simulink model "VMC_14Dof_2024a"  (R2024a)
settings: Solver=FixedStepDiscrete  StartTime=0.0  StopTime=10.0  FixedStep=0.001  RelTol=1e-3
InitFcn:
  | unlinear_14DOF_Parameters
undefined symbols (not defined in the file): Bf, Br, Cp_fl, Cp_fr, Cp_rl, Cp_rr, Cs_f, eta_FMotor, eta_RMotor, f, g, He, Hp, i_fa, i_ra, i_sw, I_tire, Ix, Iy, Iz, ks_f, kw, Lf, Lr, m, mb, mu, mw, r, Sampletime, Standstill_buffer, vx0, vxlim, w0
libraries: simulink x32, slpidlib x6
(part 4 of 5)

== system VMC_14Dof_2024a/Subsystem/Body/global system transform/integrator2 ==
  In : Inport
  Add : Sum
  Add1 : Sum
  Constant : Constant  Value=Sampletime  OutDataTypeStr=single
  Constant1 : Constant  Value=0  OutDataTypeStr=single
  Delay1 : Delay  DelayLength=1  InitialCondition=0
  Divide : Product  Inputs=**
  Out : Outport  VectorParamsAs1DForOutWhenUnconnected=off
  wires:
  In/1 -> Divide/1
  Constant/1 -> Divide/2
  Divide/1 -> Add/1
  Delay1/1 -> Add/2, Add1/2
  Constant1/1 -> Add1/1
  Add/1 -> Delay1/1
  Add1/1 -> Out/1

== system VMC_14Dof_2024a/Subsystem/Body/global system transform/integrator8 ==
  wz : Inport
  Add : Sum
  Add1 : Sum
  Constant : Constant  Value=Sampletime  OutDataTypeStr=single
  Constant1 : Constant  Value=0  OutDataTypeStr=single
  Delay1 : Delay  DelayLength=1  InitialCondition=0
  Divide : Product  Inputs=**
  Out : Outport  VectorParamsAs1DForOutWhenUnconnected=off
  wires:
  wz/1 -> Divide/1
  Constant/1 -> Divide/2
  Divide/1 -> Add/1
  Delay1/1 -> Add/2, Add1/2
  Constant1/1 -> Add1/1
  Add/1 -> Delay1/1
  Add1/1 -> Out/1

== system VMC_14Dof_2024a/Subsystem/Wheel/fl/integrator ==
  In : Inport
  Add : Sum
  Add1 : Sum
  Constant : Constant  Value=Sampletime  OutDataTypeStr=single
  Constant1 : Constant  Value=w0  OutDataTypeStr=single
  Delay1 : Delay  DelayLength=1  InitialCondition=0
  Divide : Product  Inputs=**
  Out : Outport  VectorParamsAs1DForOutWhenUnconnected=off
  wires:
  In/1 -> Divide/1
  Constant/1 -> Divide/2
  Divide/1 -> Add/1
  Delay1/1 -> Add/2, Add1/2
  Constant1/1 -> Add1/1
  Add/1 -> Delay1/1
  Add1/1 -> Out/1

== system VMC_14Dof_2024a/Subsystem/Wheel/fr/integrator ==
  In : Inport
  Add : Sum
  Add1 : Sum
  Constant : Constant  Value=Sampletime  OutDataTypeStr=single
  Constant1 : Constant  Value=w0  OutDataTypeStr=single
  Delay1 : Delay  DelayLength=1  InitialCondition=0
  Divide : Product  Inputs=**
  Out : Outport  VectorParamsAs1DForOutWhenUnconnected=off
  wires:
  In/1 -> Divide/1
  Constant/1 -> Divide/2
  Divide/1 -> Add/1
  Delay1/1 -> Add/2, Add1/2
  Constant1/1 -> Add1/1
  Add/1 -> Delay1/1
  Add1/1 -> Out/1

== system VMC_14Dof_2024a/Subsystem/Wheel/rl/integrator ==
  In : Inport
  Add : Sum
  Add1 : Sum
  Constant : Constant  Value=Sampletime  OutDataTypeStr=single
  Constant1 : Constant  Value=w0  OutDataTypeStr=single
  Delay1 : Delay  DelayLength=1  InitialCondition=0
  Divide : Product  Inputs=**
  Out : Outport  VectorParamsAs1DForOutWhenUnconnected=off
  wires:
  In/1 -> Divide/1
  Constant/1 -> Divide/2
  Divide/1 -> Add/1
  Delay1/1 -> Add/2, Add1/2
  Constant1/1 -> Add1/1
  Add/1 -> Delay1/1
  Add1/1 -> Out/1

== system VMC_14Dof_2024a/Subsystem/Wheel/rr/integrator ==
  In : Inport
  Add : Sum
  Add1 : Sum
  Constant : Constant  Value=Sampletime  OutDataTypeStr=single
  Constant1 : Constant  Value=w0  OutDataTypeStr=single
  Delay1 : Delay  DelayLength=1  InitialCondition=0
  Divide : Product  Inputs=**
  Out : Outport  VectorParamsAs1DForOutWhenUnconnected=off
  wires:
  In/1 -> Divide/1
  Constant/1 -> Divide/2
  Divide/1 -> Add/1
  Delay1/1 -> Add/2, Add1/2
  Constant1/1 -> Add1/1
  Add/1 -> Delay1/1
  Add1/1 -> Out/1

== system VMC_14Dof_2024a/Subsystem/alpha_lamda/alpha/fl ==
  vx : Inport
  vy : Inport  Port=2
  wz : Inport  Port=3
  delta_fl : Inport  Port=4
  Add2 : Sum
  Add3 : Sum  Inputs=+-
  Add4 : Sum  Inputs=-+
  Divide : Product  Inputs=/*
  Gain3 : Gain  Gain=Lf
  Gain4 : Gain  Gain=0.5*Bf
  Trigonometric Function : Trigonometry  Operator=atan
  alpha_fl : Outport  VectorParamsAs1DForOutWhenUnconnected=off
  wires:
  Gain3/1 -> Add2/2
  Gain4/1 -> Add3/2
  Add2/1 -> Divide/2
  Add3/1 -> Divide/1
  Divide/1 -> Trigonometric Function/1
  Trigonometric Function/1 -> Add4/1
  vx/1 -> Add3/1
  delta_fl/1 -> Add4/2
  vy/1 -> Add2/1
  Add4/1 -> alpha_fl/1
  wz/1 -> Gain4/1, Gain3/1

== system VMC_14Dof_2024a/Subsystem/alpha_lamda/alpha/fr ==
  vx : Inport
  vy : Inport  Port=2
  wz : Inport  Port=3
  delta_fr : Inport  Port=4
  Add2 : Sum
  Add3 : Sum
  Add4 : Sum  Inputs=-+
  Divide : Product  Inputs=/*
  Gain3 : Gain  Gain=Lf
  Gain4 : Gain  Gain=0.5*Bf
  Trigonometric Function : Trigonometry  Operator=atan
  alpha_fr : Outport  VectorParamsAs1DForOutWhenUnconnected=off
  wires:
  Gain4/1 -> Add3/2
  wz/1 -> Gain3/1, Gain4/1
  Add4/1 -> alpha_fr/1
  vy/1 -> Add2/1
  delta_fr/1 -> Add4/2
  vx/1 -> Add3/1
  Trigonometric Function/1 -> Add4/1
  Divide/1 -> Trigonometric Function/1
  Add3/1 -> Divide/1
  Add2/1 -> Divide/2
  Gain3/1 -> Add2/2

== system VMC_14Dof_2024a/Subsystem/alpha_lamda/alpha/rl ==
  vx : Inport
  vy : Inport  Port=2
  wz : Inport  Port=3
  Add2 : Sum  Inputs=+-
  Add3 : Sum  Inputs=+-
  Divide : Product  Inputs=/*
  Gain1 : Gain  Gain=-1
  Gain3 : Gain  Gain=Lr
  Gain4 : Gain  Gain=0.5*Br
  Trigonometric Function : Trigonometry  Operator=atan
  alpha_rl : Outport  VectorParamsAs1DForOutWhenUnconnected=off
  wires:
  Gain1/1 -> alpha_rl/1
  Gain4/1 -> Add3/2
  Trigonometric Function/1 -> Gain1/1
  wz/1 -> Gain3/1, Gain4/1
  vy/1 -> Add2/1
  vx/1 -> Add3/1
  Divide/1 -> Trigonometric Function/1
  Add3/1 -> Divide/1
  Add2/1 -> Divide/2
  Gain3/1 -> Add2/2

== system VMC_14Dof_2024a/Subsystem/alpha_lamda/alpha/rr ==
  vx : Inport
  vy : Inport  Port=2
  wz : Inport  Port=3
  Add2 : Sum  Inputs=+-
  Add3 : Sum
  Divide : Product  Inputs=/*
  Gain2 : Gain  Gain=-1
  Gain3 : Gain  Gain=Lr
  Gain4 : Gain  Gain=0.5*Br
  Trigonometric Function : Trigonometry  Operator=atan
  alpha_rr : Outport  VectorParamsAs1DForOutWhenUnconnected=off
  wires:
  Gain2/1 -> alpha_rr/1
  Gain4/1 -> Add3/2
  Gain3/1 -> Add2/2
  Add2/1 -> Divide/2
  Add3/1 -> Divide/1
  Divide/1 -> Trigonometric Function/1
  vx/1 -> Add3/1
  vy/1 -> Add2/1
  wz/1 -> Gain4/1, Gain3/1
  Trigonometric Function/1 -> Gain2/1

== system VMC_14Dof_2024a/Subsystem/alpha_lamda/lamda/fl ==
  w_fl : Inport
  wz : Inport  Port=2
  vx : Inport  Port=3
  vy : Inport  Port=4
  delta_fl : Inport  Port=5
  Add1 : Sum  Inputs=-+
  Add2 : Sum
  Add3 : Sum
  Add4 : Sum  Inputs=+-
  Constant1 : Constant  Value=r  OutDataTypeStr=single
  Divide1 : Product  Inputs=**
  Divide2 : Product  Inputs=**
  Divide3 : Product  Inputs=**
  Divide4 : Product  Inputs=/*
  Divide5 : Product  Inputs=*/
  Fcn1 : Fcn  Expr=u+(u==0)*eps
  Gain2 : Gain  Gain=0.5*Bf
  Gain3 : Gain  Gain=Lf
  Saturation : Saturate  UpperLimit=1  LowerLimit=-1
  Switch : Switch  Criteria=u2 > Threshold  SaturateOnIntegerOverflow=off  InputSameDT=off
  Trigonometric Function1 : Trigonometry
  Trigonometric Function2 : Trigonometry  Operator=cos
  lamda_fl : Outport  VectorParamsAs1DForOutWhenUnconnected=off
  wires:
  Saturation/1 -> lamda_fl/1
  Divide3/1 -> Fcn1/1, Add4/1  "w*I_tire"
  Constant1/1 -> Divide3/2
  w_fl/1 -> Divide3/1
  Divide2/1 -> Add3/2
  Divide1/1 -> Add3/1
  Trigonometric Function1/1 -> Divide2/2
  Add2/1 -> Divide2/1
  Gain3/1 -> Add2/1
  vy/1 -> Add2/2
  Trigonometric Function2/1 -> Divide1/2
  delta_fl/1 -> Trigonometric Function1/1, Trigonometric Function2/1
  Add1/1 -> Divide1/1
  wz/1 -> Gain2/1, Gain3/1
  Gain2/1 -> Add1/1
  vx/1 -> Add1/2
  Fcn1/1 -> Divide4/1
  Divide5/1 -> Switch/3
  Divide4/1 -> Switch/1
  Add4/1 -> Divide5/1, Divide4/2, Switch/2
  Add3/1 -> Divide5/2, Add4/2  "Vwx_fl"
  Switch/1 -> Saturation/1

== system VMC_14Dof_2024a/Subsystem/alpha_lamda/lamda/fr ==
  w_fr : Inport
  wz : Inport  Port=2
  vx : Inport  Port=3
  vy : Inport  Port=4
  delta_fr : Inport  Port=5
  Add1 : Sum
  Add2 : Sum
  Add3 : Sum
  Add4 : Sum  Inputs=+-
  Constant1 : Constant  Value=r  OutDataTypeStr=single
  Divide1 : Product  Inputs=**
  Divide2 : Product  Inputs=**
  Divide3 : Product  Inputs=**
  Divide4 : Product  Inputs=/*
  Divide5 : Product  Inputs=*/
  Fcn1 : Fcn  Expr=u+(u==0)*eps
  Gain2 : Gain  Gain=0.5*Bf
  Gain3 : Gain  Gain=Lf
  Saturation : Saturate  UpperLimit=1  LowerLimit=-1
  Switch : Switch  Criteria=u2 > Threshold  SaturateOnIntegerOverflow=off  InputSameDT=off
  Trigonometric Function1 : Trigonometry
  Trigonometric Function2 : Trigonometry  Operator=cos
  lamda_fr : Outport  VectorParamsAs1DForOutWhenUnconnected=off
  wires:
  Switch/1 -> Saturation/1
  Add3/1 -> Add4/2, Divide5/2  "Vwx_fr"
  Add4/1 -> Switch/2, Divide4/2, Divide5/1
  Divide4/1 -> Switch/1
  Divide5/1 -> Switch/3
  Fcn1/1 -> Divide4/1
  Divide3/1 -> Add4/1, Fcn1/1  "w*I_tire"
  Constant1/1 -> Divide3/2
  w_fr/1 -> Divide3/1
  Divide2/1 -> Add3/2
  Divide1/1 -> Add3/1
  Trigonometric Function1/1 -> Divide2/2
  Add2/1 -> Divide2/1
  Gain3/1 -> Add2/1
  vy/1 -> Add2/2
  Trigonometric Function2/1 -> Divide1/2
  delta_fr/1 -> Trigonometric Function1/1, Trigonometric Function2/1
  Add1/1 -> Divide1/1
  wz/1 -> Gain2/1, Gain3/1
  Gain2/1 -> Add1/1
  vx/1 -> Add1/2
  Saturation/1 -> lamda_fr/1

== system VMC_14Dof_2024a/Subsystem/alpha_lamda/lamda/rl ==
  w_rl : Inport
  wz : Inport  Port=2
  vx : Inport  Port=3
  Add1 : Sum  Inputs=-+
  Add4 : Sum  Inputs=+-
  Constant1 : Constant  Value=r  OutDataTypeStr=single
  Divide3 : Product  Inputs=**
  Divide4 : Product  Inputs=/*
  Divide5 : Product  Inputs=*/
  Fcn1 : Fcn  Expr=u+(u==0)*eps
  Gain2 : Gain  Gain=0.5*Br
  Saturation : Saturate  UpperLimit=1  LowerLimit=-1
  Switch : Switch  Criteria=u2 > Threshold  SaturateOnIntegerOverflow=off  InputSameDT=off
  lamda_rl : Outport  VectorParamsAs1DForOutWhenUnconnected=off
  wires:
  Switch/1 -> Saturation/1
  Add1/1 -> Add4/2, Divide5/2
  Add4/1 -> Switch/2, Divide4/2, Divide5/1
  Divide4/1 -> Switch/1
  Divide5/1 -> Switch/3
  Fcn1/1 -> Divide4/1
  Divide3/1 -> Add4/1, Fcn1/1  "w*I_tire"
  Constant1/1 -> Divide3/2
  w_rl/1 -> Divide3/1
  wz/1 -> Gain2/1
  Gain2/1 -> Add1/1
  vx/1 -> Add1/2
  Saturation/1 -> lamda_rl/1

== system VMC_14Dof_2024a/Subsystem/alpha_lamda/lamda/rr ==
  w_rr : Inport
  wz : Inport  Port=2
  vx : Inport  Port=3
  Add1 : Sum
  Add4 : Sum  Inputs=+-
  Constant1 : Constant  Value=r  OutDataTypeStr=single
  Divide3 : Product  Inputs=**
  Divide4 : Product  Inputs=/*
  Divide5 : Product  Inputs=*/
  Fcn1 : Fcn  Expr=u+(u==0)*eps
  Gain2 : Gain  Gain=0.5*Br
  Saturation : Saturate  UpperLimit=1  LowerLimit=-1
  Switch : Switch  Criteria=u2 > Threshold  SaturateOnIntegerOverflow=off  InputSameDT=off
  lamda_rr : Outport  VectorParamsAs1DForOutWhenUnconnected=off
  wires:
  Add1/1 -> Add4/2, Divide5/2  "Vwx_rr"
  Add4/1 -> Switch/2, Divide4/2, Divide5/1
  Divide4/1 -> Switch/1
  Divide5/1 -> Switch/3
  Fcn1/1 -> Divide4/1
  Divide3/1 -> Add4/1, Fcn1/1  "w*I_tire"
  vx/1 -> Add1/2
  Gain2/1 -> Add1/1
  wz/1 -> Gain2/1
  w_rr/1 -> Divide3/1
  Constant1/1 -> Divide3/2
  Switch/1 -> Saturation/1
  Saturation/1 -> lamda_rr/1

== system VMC_14Dof_2024a/Subsystem1/Traction_Control/LSD_Enable/LSD_EnableFL ==
  BrkDmd : Inport
  WhlSpdActlFL : Inport  Port=2
  WhlSpdRefFL : Inport  Port=3
  Compare To Constant1 : simulink/Logic and Bit Operations/Compare To Constant  relop=<  const=0.1  OutDataTypeStr=boolean
  Compare To Constant3 : simulink/Logic and Bit Operations/Compare To Constant  relop=>=  const=2  OutDataTypeStr=boolean
  Logical Operator : Logic  Inputs=3  AllPortsSameDT=off  OutDataTypeStr=boolean
  SlipJudge : simulink/Logic and Bit Operations/Compare To Constant  relop=>=  const=0.1  OutDataTypeStr=boolean
  LSD_EnableFL : Outport  VectorParamsAs1DForOutWhenUnconnected=off
  wires:
  WhlSpdActlFL/1 -> Compare To Constant3/1
  WhlSpdRefFL/1 -> SlipJudge/1  "SlipRateFL"
  Compare To Constant1/1 -> Logical Operator/1
  BrkDmd/1 -> Compare To Constant1/1
  Logical Operator/1 -> LSD_EnableFL/1  "LSD_EnableFL"
  Compare To Constant3/1 -> Logical Operator/2
  SlipJudge/1 -> Logical Operator/3

== system VMC_14Dof_2024a/Subsystem1/Traction_Control/LSD_Enable/LSD_EnableFR ==
  BrkDmd : Inport
  WhlSpdActlFR : Inport  Port=2
  WhlSpdRefFR : Inport  Port=3
  Compare To Constant1 : simulink/Logic and Bit Operations/Compare To Constant  relop=<  const=0.1  OutDataTypeStr=boolean
  Compare To Constant3 : simulink/Logic and Bit Operations/Compare To Constant  relop=>=  const=2  OutDataTypeStr=boolean
  Logical Operator : Logic  Inputs=3  AllPortsSameDT=off  OutDataTypeStr=boolean
  SlipJudge : simulink/Logic and Bit Operations/Compare To Constant  relop=>=  const=0.1  OutDataTypeStr=boolean
  LSD_EnableFL : Outport  VectorParamsAs1DForOutWhenUnconnected=off
  wires:
  SlipJudge/1 -> Logical Operator/3
  Compare To Constant3/1 -> Logical Operator/2
  Logical Operator/1 -> LSD_EnableFL/1  "LSD_EnableFL"
  BrkDmd/1 -> Compare To Constant1/1
  Compare To Constant1/1 -> Logical Operator/1
  WhlSpdRefFR/1 -> SlipJudge/1  "SlipRateFR"
  WhlSpdActlFR/1 -> Compare To Constant3/1

== system VMC_14Dof_2024a/Subsystem1/Traction_Control/LSD_Enable/LSD_EnableRL ==
  BrkDmd : Inport
  WhlSpdActlRL : Inport  Port=2
  WhlSpdRefRL : Inport  Port=3
  Compare To Constant1 : simulink/Logic and Bit Operations/Compare To Constant  relop=<  const=0.1  OutDataTypeStr=boolean
  Compare To Constant3 : simulink/Logic and Bit Operations/Compare To Constant  relop=>=  const=2  OutDataTypeStr=boolean
  Logical Operator : Logic  Inputs=3  AllPortsSameDT=off  OutDataTypeStr=boolean
  SlipJudge : simulink/Logic and Bit Operations/Compare To Constant  relop=>=  const=0.1  OutDataTypeStr=boolean
  LSD_EnableFL : Outport  VectorParamsAs1DForOutWhenUnconnected=off
  wires:
  WhlSpdActlRL/1 -> Compare To Constant3/1
  WhlSpdRefRL/1 -> SlipJudge/1  "SlipRateRL"
  Compare To Constant1/1 -> Logical Operator/1
  BrkDmd/1 -> Compare To Constant1/1
  Logical Operator/1 -> LSD_EnableFL/1  "LSD_EnableFL"
  Compare To Constant3/1 -> Logical Operator/2
  SlipJudge/1 -> Logical Operator/3

== system VMC_14Dof_2024a/Subsystem1/Traction_Control/LSD_Enable/LSD_EnableRR  ==
  BrkDmd : Inport
  WhlSpdActlRR : Inport  Port=2
  WhlSpdRefRR : Inport  Port=3
  Compare To Constant1 : simulink/Logic and Bit Operations/Compare To Constant  relop=<  const=0.1  OutDataTypeStr=boolean
  Compare To Constant3 : simulink/Logic and Bit Operations/Compare To Constant  relop=>=  const=2  OutDataTypeStr=boolean
  Logical Operator : Logic  Inputs=3  AllPortsSameDT=off  OutDataTypeStr=boolean
  SlipJudge : simulink/Logic and Bit Operations/Compare To Constant  relop=>=  const=0.1  OutDataTypeStr=boolean
  LSD_EnableFL : Outport  VectorParamsAs1DForOutWhenUnconnected=off
  wires:
  SlipJudge/1 -> Logical Operator/3
  Compare To Constant3/1 -> Logical Operator/2
  Logical Operator/1 -> LSD_EnableFL/1  "LSD_EnableFL"
  BrkDmd/1 -> Compare To Constant1/1
  Compare To Constant1/1 -> Logical Operator/1
  WhlSpdRefRR/1 -> SlipJudge/1  "SlipRateRR"
  WhlSpdActlRR/1 -> Compare To Constant3/1

== system VMC_14Dof_2024a/Subsystem1/Traction_Control/LimitedSlipDifferential/LSD_Ctrl ==
  Vehicle_States : Inport
  LSD_Enable : Inport  Port=2
  Bus Creator{,1..3} (4 alike) : BusCreator  Inputs=3
  Bus Selector : BusSelector  OutputSignals=Wheel.Ref_WheelSpeed_Array_radps,Vehicle_Static_Parameter.Gear_Ratio_NA,Torque_Demand.MotorSpeed_Array_rpm
  Constant : Constant  Value=30 / pi  OutDataTypeStr=single
  Demux : Demux
  Demux1 : Demux
  Demux2 : Demux
  Divide : Product  Inputs=***  OutDataTypeStr=single
  LSD_CtrlFL : Outport
  LSD_CtrlFR : Outport  Port=2
  LSD_CtrlRL : Outport  Port=3
  LSD_CtrlRR : Outport  Port=4
  wires:
  Constant/1 -> Divide/3
  Demux2/4 -> Bus Creator3/1  "MotSpdRefByrpmRR"
  Divide/1 -> Demux2/1  "MotSpdRefbyrpm"
  Demux2/1 -> Bus Creator/1  "MotSpdRefByrpmFL"
  Demux2/2 -> Bus Creator1/1  "MotSpdRefByrpmFR"
  Demux2/3 -> Bus Creator2/1  "MotSpdRefByrpmRL"
  Demux1/4 -> Bus Creator3/2  "MotSpdActlByrpmRR"
  Demux1/2 -> Bus Creator1/2  "MotSpdActlByrpmFR"
  Demux1/3 -> Bus Creator2/2  "MotSpdActlByrpmRL"
  Demux1/1 -> Bus Creator/2  "MotSpdActlByrpmFL"
  Demux/1 -> Bus Creator/3  "LSD_EnableFL"
  Demux/2 -> Bus Creator1/3  "LSD_EnableFR"
  Demux/3 -> Bus Creator2/3  "LSD_EnableRL"
  Demux/4 -> Bus Creator3/3  "LSD_EnableRR"
  Bus Creator/1 -> LSD_CtrlFL/1  "LSD_CtrlFL"
  Bus Creator1/1 -> LSD_CtrlFR/1  "LSD_CtrlFR"
  Bus Creator2/1 -> LSD_CtrlRL/1  "LSD_CtrlRL"
  Bus Creator3/1 -> LSD_CtrlRR/1  "LSD_CtrlRR"
  Bus Selector/1 -> Divide/1  "<Ref_WheelSpeed_Array_radps>"
  LSD_Enable/1 -> Demux/1
  Bus Selector/3 -> Demux1/1  "<MotorSpeed_Array_rpm>"
  Vehicle_States/1 -> Bus Selector/1
  Bus Selector/2 -> Divide/2  "<Gear_Ratio_NA>"

== system VMC_14Dof_2024a/Subsystem1/Traction_Control/LimitedSlipDifferential/PID_CtrlFL ==
  LSD_CtrlFL : Inport
  EDS_TrqFL : Inport  Port=2
  PID_Setting : Inport  Port=3
  Add1 : Sum  AccumDataTypeStr=single
  Bus Selector : BusSelector  OutputSignals=MotSpdRefByrpmFL,MotSpdActlByrpmFL,LSD_EnableFL
  Demux : Demux  Outputs=5
  Gain : Gain  Gain=0.001  ParamDataTypeStr=single  OutDataTypeStr=single
  PID Controller : slpidlib/PID Controller  Controller=PID  Form=Parallel  TimeDomain=Discrete-time  UseExternalTs=off  SampleTime=-1  IntegratorMethod=Forward Euler  FilterMethod=Forward Euler  ControllerParametersSource=external  P=500  I=0  UseKiTs=off  D=0  UseExternalDerivativeSource=off  N=100  UseFilter=on  TunerSelectOption=Transfer Function Based (PID Tuner App)  InitialConditionSource=internal  InitialConditionForIntegrator=0  InitialConditionForFilter=0  DifferentiatorICPrevScaledInput=0  ExternalReset=rising  TrackingMode=off  Kt=1  LimitOutput=off  SatLimitsSource=internal  UpperSaturationLimit=inf  LowerSaturationLimit=-inf  LinearizeAsGain=on  AntiWindupMode=none  Kb=1  LimitIntegrator=off  UpperIntegratorSaturationLimit=inf  LowerIntegratorSaturationLimit=-inf  PGainOutDataTypeStr=single  PProdOutDataTypeStr=single  POutMin=[]  POutMax=[]  IGainOutDataTypeStr=single  IProdOutDataTypeStr=single  IOutMin=[]  IOutMax=[]  DGainOutDataTypeStr=single  DProdOutDataTypeStr=single  DOutMin=[]  DOutMax=[]  NGainOutDataTypeStr=single  NProdOutDataTypeStr=single  NOutMin=[]  NOutMax=[]  SumOutDataTypeStr=single  SumOutMin=[]  SumOutMax=[]  SaturationOutMin=[]  SaturationOutMax=[]  PParamMin=[]  PParamMax=[]  IParamMin=[]  IParamMax=[]  DParamMin=[]  DParamMax=[]  NParamMin=[]  NParamMax=[]  KbParamMin=[]  KbParamMax=[]  KtParamMin=[]  KtParamMax=[]  KbOutMin=[]  KbOutMax=[]  KtOutMin=[]  KtOutMax=[]  IntegratorOutMin=[]  IntegratorOutMax=[]  FilterOutMin=[]  FilterOutMax=[]  SumI1OutMin=[]  SumI1OutMax=[]  SumI2OutMin=[]  SumI2OutMax=[]  SumI3OutMin=[]  SumI3OutMax=[]  SumI4OutMin=[]  SumI4OutMax=[]  SumDOutMin=[]  SumDOutMax=[]  DifferentiatorOutMin=[]  DifferentiatorOutMax=[]  FilterDiffOutCoefMin=[]  FilterDiffOutCoefMax=[]  ReciprocalOutMin=[]  ReciprocalOutMax=[]  SumDenOutMin=[]  SumDenOutMax=[]  SumNumOutMin=[]  SumNumOutMax=[]  DivideOutMin=[]  DivideOutMax=[]  UdiffTsProdOutMin=[]  UdiffTsProdOutMax=[]  NTsProdOutMin=[]  NTsProdOutMax=[]  UintegralTsProdOutMin=[]  UintegralTsProdOutMax=[]  UngainTsProdOutMin=[]  UngainTsProdOutMax=[]  ClampingZeroOutDataTypeStr=Inherit: Inherit via back propagation  ClampingZeroOutMin=[]  ClampingZeroOutMax=[]  FilterDenConstantOutDataTypeStr=Inherit: Inherit via back propagation  FilterDenConstantOutMin=[]  FilterDenConstantOutMax=[]  PCopyOutDataTypeStr=Inherit: Inherit via back propagation  PCopyOutMin=[]  PCopyOutMax=[]  NCopyOutDataTypeStr=Inherit: Inherit via back propagation  NCopyOutMin=[]  NCopyOutMax=[]  IntegratorContinuousStateAttributes=''  IntegratorStateMustResolveToSignalObject=off  IntegratorRTWStateStorageClass=Auto  FilterContinuousStateAttributes=''  FilterStateMustResolveToSignalObject=off  FilterRTWStateStorageClass=Auto  ParallelPVariant=ExternalParameters  IdealPVariant=Disabled  IVariant=ExternalParameters  DVariant=ExternalParameters  IntegratorVariant=Discrete  SatVariant=Disabled  AWVariant=Passthrough  PCopyVariant=Disabled  TRVariant=Disabled  FdbkBlocksVariant=Forward  IdealPFdbkVariant=Disabled  SatFdbkVariant=Disabled  DerivativeFilterVariant=ForwardEulerFilter  NVariant=ExternalParameters  NCopyVariant=Disabled  FilterICVariant=InternalICsFilter  IntegratorICVariant=InternalICs  ExternalResetVariant=ExternalReset  TRSumVariant=Passthrough  SumFdbkVariant=Disabled  SumVariant=Sum_PID  TsampFilterVariant=InternalTs  TsampNgainVariant=Passthrough  TsampIntegralVariant=Disabled_SignalSpec  ExternalSaturationOutDataTypeStr=Inherit: Same as second input  DerivativeSourceVariant=ErrorSignal
  Saturation1 : Saturate  UpperLimit=0  LowerLimit=-10
  SpdDiffFL : Sum  Inputs=+-  OutDataTypeStr=single  AccumDataTypeStr=single
  Switch : Switch  Criteria=u2 > Threshold  OutDataTypeStr=single  SaturateOnIntegerOverflow=off  InputSameDT=off
  LSD_TrqFL : Outport  VectorParamsAs1DForOutWhenUnconnected=off
  wires:
  Add1/1 -> Switch/1  "LSDTrqFL"
  EDS_TrqFL/1 -> Add1/2, Switch/3
  LSD_CtrlFL/1 -> Bus Selector/1
  Bus Selector/1 -> SpdDiffFL/1  "<MotSpdRefByrpmFL>"
  Bus Selector/2 -> SpdDiffFL/2  "<MotSpdActlByrpmFL>"
  Bus Selector/3 -> Switch/2  "<LSD_EnableFL>"
  Switch/1 -> LSD_TrqFL/1  "LSD_TrqFL"
  Demux/4 -> PID Controller/5  "N"
  Demux/1 -> PID Controller/2  "P"
  PID Controller/1 -> Saturation1/1  "TrqModFL"
  Demux/2 -> PID Controller/3  "I"
  Demux/3 -> PID Controller/4  "D"
  Demux/5 -> PID Controller/6  "PID_Reset"
  PID_Setting/1 -> Demux/1
  Gain/1 -> PID Controller/1  "SpdDiffFLScaled"
  SpdDiffFL/1 -> Gain/1  "SpdDiffFL"
  Saturation1/1 -> Add1/1

== system VMC_14Dof_2024a/Subsystem1/Traction_Control/LimitedSlipDifferential/PID_CtrlFR ==
  LSD_CtrlFR : Inport
  EDS_TrqFR : Inport  Port=2
  PID_Setting : Inport  Port=3
  Add1 : Sum  AccumDataTypeStr=single
  Bus Selector : BusSelector  OutputSignals=MotSpdRefByrpmFR,MotSpdActlByrpmFR,LSD_EnableFR
  Demux : Demux  Outputs=5
  Gain : Gain  Gain=0.001  ParamDataTypeStr=single  OutDataTypeStr=single
  PID Controller : slpidlib/PID Controller  Controller=PID  Form=Parallel  TimeDomain=Discrete-time  UseExternalTs=off  SampleTime=-1  IntegratorMethod=Forward Euler  FilterMethod=Forward Euler  ControllerParametersSource=external  P=500  I=0  UseKiTs=off  D=0  UseExternalDerivativeSource=off  N=100  UseFilter=on  TunerSelectOption=Transfer Function Based (PID Tuner App)  InitialConditionSource=internal  InitialConditionForIntegrator=0  InitialConditionForFilter=0  DifferentiatorICPrevScaledInput=0  ExternalReset=rising  TrackingMode=off  Kt=1  LimitOutput=off  SatLimitsSource=internal  UpperSaturationLimit=inf  LowerSaturationLimit=-inf  LinearizeAsGain=on  AntiWindupMode=none  Kb=1  LimitIntegrator=off  UpperIntegratorSaturationLimit=inf  LowerIntegratorSaturationLimit=-inf  PGainOutDataTypeStr=single  PProdOutDataTypeStr=single  POutMin=[]  POutMax=[]  IGainOutDataTypeStr=single  IProdOutDataTypeStr=single  IOutMin=[]  IOutMax=[]  DGainOutDataTypeStr=single  DProdOutDataTypeStr=single  DOutMin=[]  DOutMax=[]  NGainOutDataTypeStr=single  NProdOutDataTypeStr=single  NOutMin=[]  NOutMax=[]  SumOutDataTypeStr=single  SumOutMin=[]  SumOutMax=[]  SaturationOutMin=[]  SaturationOutMax=[]  PParamMin=[]  PParamMax=[]  IParamMin=[]  IParamMax=[]  DParamMin=[]  DParamMax=[]  NParamMin=[]  NParamMax=[]  KbParamMin=[]  KbParamMax=[]  KtParamMin=[]  KtParamMax=[]  KbOutMin=[]  KbOutMax=[]  KtOutMin=[]  KtOutMax=[]  IntegratorOutMin=[]  IntegratorOutMax=[]  FilterOutMin=[]  FilterOutMax=[]  SumI1OutMin=[]  SumI1OutMax=[]  SumI2OutMin=[]  SumI2OutMax=[]  SumI3OutMin=[]  SumI3OutMax=[]  SumI4OutMin=[]  SumI4OutMax=[]  SumDOutMin=[]  SumDOutMax=[]  DifferentiatorOutMin=[]  DifferentiatorOutMax=[]  FilterDiffOutCoefMin=[]  FilterDiffOutCoefMax=[]  ReciprocalOutMin=[]  ReciprocalOutMax=[]  SumDenOutMin=[]  SumDenOutMax=[]  SumNumOutMin=[]  SumNumOutMax=[]  DivideOutMin=[]  DivideOutMax=[]  UdiffTsProdOutMin=[]  UdiffTsProdOutMax=[]  NTsProdOutMin=[]  NTsProdOutMax=[]  UintegralTsProdOutMin=[]  UintegralTsProdOutMax=[]  UngainTsProdOutMin=[]  UngainTsProdOutMax=[]  ClampingZeroOutDataTypeStr=Inherit: Inherit via back propagation  ClampingZeroOutMin=[]  ClampingZeroOutMax=[]  FilterDenConstantOutDataTypeStr=Inherit: Inherit via back propagation  FilterDenConstantOutMin=[]  FilterDenConstantOutMax=[]  PCopyOutDataTypeStr=Inherit: Inherit via back propagation  PCopyOutMin=[]  PCopyOutMax=[]  NCopyOutDataTypeStr=Inherit: Inherit via back propagation  NCopyOutMin=[]  NCopyOutMax=[]  IntegratorContinuousStateAttributes=''  IntegratorStateMustResolveToSignalObject=off  IntegratorRTWStateStorageClass=Auto  FilterContinuousStateAttributes=''  FilterStateMustResolveToSignalObject=off  FilterRTWStateStorageClass=Auto  ParallelPVariant=ExternalParameters  IdealPVariant=Disabled  IVariant=ExternalParameters  DVariant=ExternalParameters  IntegratorVariant=Discrete  SatVariant=Disabled  AWVariant=Passthrough  PCopyVariant=Disabled  TRVariant=Disabled  FdbkBlocksVariant=Forward  IdealPFdbkVariant=Disabled  SatFdbkVariant=Disabled  DerivativeFilterVariant=ForwardEulerFilter  NVariant=ExternalParameters  NCopyVariant=Disabled  FilterICVariant=InternalICsFilter  IntegratorICVariant=InternalICs  ExternalResetVariant=ExternalReset  TRSumVariant=Passthrough  SumFdbkVariant=Disabled  SumVariant=Sum_PID  TsampFilterVariant=InternalTs  TsampNgainVariant=Passthrough  TsampIntegralVariant=Disabled_SignalSpec  ExternalSaturationOutDataTypeStr=Inherit: Same as second input  DerivativeSourceVariant=ErrorSignal
  Saturation1 : Saturate  UpperLimit=0  LowerLimit=-10
  SpdDiffFR : Sum  Inputs=+-  OutDataTypeStr=single  AccumDataTypeStr=single
  Switch : Switch  Criteria=u2 > Threshold  OutDataTypeStr=single  SaturateOnIntegerOverflow=off  InputSameDT=off
  LSD_TrqFR : Outport  VectorParamsAs1DForOutWhenUnconnected=off
  wires:
  Add1/1 -> Switch/1  "LSDTrqFR"
  LSD_CtrlFR/1 -> Bus Selector/1
  Switch/1 -> LSD_TrqFR/1  "LSD_TrqFR"
  Bus Selector/3 -> Switch/2  "<LSD_EnableFR>"
  EDS_TrqFR/1 -> Add1/2, Switch/3
  PID Controller/1 -> Saturation1/1  "TrqModFR"
  Bus Selector/2 -> SpdDiffFR/2  "<MotSpdActlByrpmFR>"
  Demux/3 -> PID Controller/4  "D"
  Demux/2 -> PID Controller/3  "I"
  PID_Setting/1 -> Demux/1
  Demux/5 -> PID Controller/6  "PID_Reset"
  Gain/1 -> PID Controller/1  "SpdDiffFRScaled"
  Demux/4 -> PID Controller/5  "N"
  Bus Selector/1 -> SpdDiffFR/1  "<MotSpdRefByrpmFR>"
  Demux/1 -> PID Controller/2  "P"
  SpdDiffFR/1 -> Gain/1  "SpdDiffFR"
  Saturation1/1 -> Add1/1

== system VMC_14Dof_2024a/Subsystem1/Traction_Control/LimitedSlipDifferential/PID_CtrlRL ==
  LSD_CtrlRL : Inport
  EDS_TrqRL : Inport  Port=2
  PID_Setting : Inport  Port=3
  Add1 : Sum  AccumDataTypeStr=single
  Bus Selector : BusSelector  OutputSignals=MotSpdRefByrpmRL,MotSpdActlByrpmRL,LSD_EnableRL
  Demux : Demux  Outputs=5
  Gain : Gain  Gain=0.001  ParamDataTypeStr=single  OutDataTypeStr=single
  PID Controller : slpidlib/PID Controller  Controller=PID  Form=Parallel  TimeDomain=Discrete-time  UseExternalTs=off  SampleTime=-1  IntegratorMethod=Forward Euler  FilterMethod=Forward Euler  ControllerParametersSource=external  P=500  I=0  UseKiTs=off  D=0  UseExternalDerivativeSource=off  N=100  UseFilter=on  TunerSelectOption=Transfer Function Based (PID Tuner App)  InitialConditionSource=internal  InitialConditionForIntegrator=0  InitialConditionForFilter=0  DifferentiatorICPrevScaledInput=0  ExternalReset=rising  TrackingMode=off  Kt=1  LimitOutput=off  SatLimitsSource=internal  UpperSaturationLimit=inf  LowerSaturationLimit=-inf  LinearizeAsGain=on  AntiWindupMode=none  Kb=1  LimitIntegrator=off  UpperIntegratorSaturationLimit=inf  LowerIntegratorSaturationLimit=-inf  PGainOutDataTypeStr=single  PProdOutDataTypeStr=single  POutMin=[]  POutMax=[]  IGainOutDataTypeStr=single  IProdOutDataTypeStr=single  IOutMin=[]  IOutMax=[]  DGainOutDataTypeStr=single  DProdOutDataTypeStr=single  DOutMin=[]  DOutMax=[]  NGainOutDataTypeStr=single  NProdOutDataTypeStr=single  NOutMin=[]  NOutMax=[]  SumOutDataTypeStr=single  SumOutMin=[]  SumOutMax=[]  SaturationOutMin=[]  SaturationOutMax=[]  PParamMin=[]  PParamMax=[]  IParamMin=[]  IParamMax=[]  DParamMin=[]  DParamMax=[]  NParamMin=[]  NParamMax=[]  KbParamMin=[]  KbParamMax=[]  KtParamMin=[]  KtParamMax=[]  KbOutMin=[]  KbOutMax=[]  KtOutMin=[]  KtOutMax=[]  IntegratorOutMin=[]  IntegratorOutMax=[]  FilterOutMin=[]  FilterOutMax=[]  SumI1OutMin=[]  SumI1OutMax=[]  SumI2OutMin=[]  SumI2OutMax=[]  SumI3OutMin=[]  SumI3OutMax=[]  SumI4OutMin=[]  SumI4OutMax=[]  SumDOutMin=[]  SumDOutMax=[]  DifferentiatorOutMin=[]  DifferentiatorOutMax=[]  FilterDiffOutCoefMin=[]  FilterDiffOutCoefMax=[]  ReciprocalOutMin=[]  ReciprocalOutMax=[]  SumDenOutMin=[]  SumDenOutMax=[]  SumNumOutMin=[]  SumNumOutMax=[]  DivideOutMin=[]  DivideOutMax=[]  UdiffTsProdOutMin=[]  UdiffTsProdOutMax=[]  NTsProdOutMin=[]  NTsProdOutMax=[]  UintegralTsProdOutMin=[]  UintegralTsProdOutMax=[]  UngainTsProdOutMin=[]  UngainTsProdOutMax=[]  ClampingZeroOutDataTypeStr=Inherit: Inherit via back propagation  ClampingZeroOutMin=[]  ClampingZeroOutMax=[]  FilterDenConstantOutDataTypeStr=Inherit: Inherit via back propagation  FilterDenConstantOutMin=[]  FilterDenConstantOutMax=[]  PCopyOutDataTypeStr=Inherit: Inherit via back propagation  PCopyOutMin=[]  PCopyOutMax=[]  NCopyOutDataTypeStr=Inherit: Inherit via back propagation  NCopyOutMin=[]  NCopyOutMax=[]  IntegratorContinuousStateAttributes=''  IntegratorStateMustResolveToSignalObject=off  IntegratorRTWStateStorageClass=Auto  FilterContinuousStateAttributes=''  FilterStateMustResolveToSignalObject=off  FilterRTWStateStorageClass=Auto  ParallelPVariant=ExternalParameters  IdealPVariant=Disabled  IVariant=ExternalParameters  DVariant=ExternalParameters  IntegratorVariant=Discrete  SatVariant=Disabled  AWVariant=Passthrough  PCopyVariant=Disabled  TRVariant=Disabled  FdbkBlocksVariant=Forward  IdealPFdbkVariant=Disabled  SatFdbkVariant=Disabled  DerivativeFilterVariant=ForwardEulerFilter  NVariant=ExternalParameters  NCopyVariant=Disabled  FilterICVariant=InternalICsFilter  IntegratorICVariant=InternalICs  ExternalResetVariant=ExternalReset  TRSumVariant=Passthrough  SumFdbkVariant=Disabled  SumVariant=Sum_PID  TsampFilterVariant=InternalTs  TsampNgainVariant=Passthrough  TsampIntegralVariant=Disabled_SignalSpec  ExternalSaturationOutDataTypeStr=Inherit: Same as second input  DerivativeSourceVariant=ErrorSignal
  Saturation1 : Saturate  UpperLimit=0  LowerLimit=-10
  SpdDiffRL : Sum  Inputs=+-  OutDataTypeStr=single  AccumDataTypeStr=single
  Switch : Switch  Criteria=u2 > Threshold  OutDataTypeStr=single  SaturateOnIntegerOverflow=off  InputSameDT=off
  LSD_TrqRL : Outport  VectorParamsAs1DForOutWhenUnconnected=off
  wires:
  Add1/1 -> Switch/1  "LSDTrqRL"
  LSD_CtrlRL/1 -> Bus Selector/1
  Switch/1 -> LSD_TrqRL/1  "LSD_TrqRL"
  Bus Selector/3 -> Switch/2  "<LSD_EnableRL>"
  EDS_TrqRL/1 -> Add1/2, Switch/3
  PID Controller/1 -> Saturation1/1  "TrqModRL"
  Bus Selector/2 -> SpdDiffRL/2  "<MotSpdActlByrpmRL>"
  Demux/3 -> PID Controller/4  "D"
  Demux/2 -> PID Controller/3  "I"
  PID_Setting/1 -> Demux/1
  Demux/5 -> PID Controller/6  "PID_Reset"
  Gain/1 -> PID Controller/1  "SpdDiffRLScaled"
  Demux/4 -> PID Controller/5  "N"
  Bus Selector/1 -> SpdDiffRL/1  "<MotSpdRefByrpmRL>"
  Demux/1 -> PID Controller/2  "P"
  SpdDiffRL/1 -> Gain/1  "SpdDiffRL"
  Saturation1/1 -> Add1/1

== system VMC_14Dof_2024a/Subsystem1/Traction_Control/LimitedSlipDifferential/PID_CtrlRR ==
  LSD_CtrlRR : Inport
  EDS_TrqRR : Inport  Port=2
  PID_Setting : Inport  Port=3
  Add1 : Sum  AccumDataTypeStr=single
  Bus Selector : BusSelector  OutputSignals=MotSpdRefByrpmRR,MotSpdActlByrpmRR,LSD_EnableRR
  Demux : Demux  Outputs=5
  Gain : Gain  Gain=0.001  ParamDataTypeStr=single  OutDataTypeStr=single
  PID Controller : slpidlib/PID Controller  Controller=PID  Form=Parallel  TimeDomain=Discrete-time  UseExternalTs=off  SampleTime=-1  IntegratorMethod=Forward Euler  FilterMethod=Forward Euler  ControllerParametersSource=external  P=500  I=0  UseKiTs=off  D=0  UseExternalDerivativeSource=off  N=100  UseFilter=on  TunerSelectOption=Transfer Function Based (PID Tuner App)  InitialConditionSource=internal  InitialConditionForIntegrator=0  InitialConditionForFilter=0  DifferentiatorICPrevScaledInput=0  ExternalReset=rising  TrackingMode=off  Kt=1  LimitOutput=off  SatLimitsSource=internal  UpperSaturationLimit=inf  LowerSaturationLimit=-inf  LinearizeAsGain=on  AntiWindupMode=none  Kb=1  LimitIntegrator=off  UpperIntegratorSaturationLimit=inf  LowerIntegratorSaturationLimit=-inf  PGainOutDataTypeStr=single  PProdOutDataTypeStr=single  POutMin=[]  POutMax=[]  IGainOutDataTypeStr=single  IProdOutDataTypeStr=single  IOutMin=[]  IOutMax=[]  DGainOutDataTypeStr=single  DProdOutDataTypeStr=single  DOutMin=[]  DOutMax=[]  NGainOutDataTypeStr=single  NProdOutDataTypeStr=single  NOutMin=[]  NOutMax=[]  SumOutDataTypeStr=single  SumOutMin=[]  SumOutMax=[]  SaturationOutMin=[]  SaturationOutMax=[]  PParamMin=[]  PParamMax=[]  IParamMin=[]  IParamMax=[]  DParamMin=[]  DParamMax=[]  NParamMin=[]  NParamMax=[]  KbParamMin=[]  KbParamMax=[]  KtParamMin=[]  KtParamMax=[]  KbOutMin=[]  KbOutMax=[]  KtOutMin=[]  KtOutMax=[]  IntegratorOutMin=[]  IntegratorOutMax=[]  FilterOutMin=[]  FilterOutMax=[]  SumI1OutMin=[]  SumI1OutMax=[]  SumI2OutMin=[]  SumI2OutMax=[]  SumI3OutMin=[]  SumI3OutMax=[]  SumI4OutMin=[]  SumI4OutMax=[]  SumDOutMin=[]  SumDOutMax=[]  DifferentiatorOutMin=[]  DifferentiatorOutMax=[]  FilterDiffOutCoefMin=[]  FilterDiffOutCoefMax=[]  ReciprocalOutMin=[]  ReciprocalOutMax=[]  SumDenOutMin=[]  SumDenOutMax=[]  SumNumOutMin=[]  SumNumOutMax=[]  DivideOutMin=[]  DivideOutMax=[]  UdiffTsProdOutMin=[]  UdiffTsProdOutMax=[]  NTsProdOutMin=[]  NTsProdOutMax=[]  UintegralTsProdOutMin=[]  UintegralTsProdOutMax=[]  UngainTsProdOutMin=[]  UngainTsProdOutMax=[]  ClampingZeroOutDataTypeStr=Inherit: Inherit via back propagation  ClampingZeroOutMin=[]  ClampingZeroOutMax=[]  FilterDenConstantOutDataTypeStr=Inherit: Inherit via back propagation  FilterDenConstantOutMin=[]  FilterDenConstantOutMax=[]  PCopyOutDataTypeStr=Inherit: Inherit via back propagation  PCopyOutMin=[]  PCopyOutMax=[]  NCopyOutDataTypeStr=Inherit: Inherit via back propagation  NCopyOutMin=[]  NCopyOutMax=[]  IntegratorContinuousStateAttributes=''  IntegratorStateMustResolveToSignalObject=off  IntegratorRTWStateStorageClass=Auto  FilterContinuousStateAttributes=''  FilterStateMustResolveToSignalObject=off  FilterRTWStateStorageClass=Auto  ParallelPVariant=ExternalParameters  IdealPVariant=Disabled  IVariant=ExternalParameters  DVariant=ExternalParameters  IntegratorVariant=Discrete  SatVariant=Disabled  AWVariant=Passthrough  PCopyVariant=Disabled  TRVariant=Disabled  FdbkBlocksVariant=Forward  IdealPFdbkVariant=Disabled  SatFdbkVariant=Disabled  DerivativeFilterVariant=ForwardEulerFilter  NVariant=ExternalParameters  NCopyVariant=Disabled  FilterICVariant=InternalICsFilter  IntegratorICVariant=InternalICs  ExternalResetVariant=ExternalReset  TRSumVariant=Passthrough  SumFdbkVariant=Disabled  SumVariant=Sum_PID  TsampFilterVariant=InternalTs  TsampNgainVariant=Passthrough  TsampIntegralVariant=Disabled_SignalSpec  ExternalSaturationOutDataTypeStr=Inherit: Same as second input  DerivativeSourceVariant=ErrorSignal
  Saturation1 : Saturate  UpperLimit=0  LowerLimit=-10
  SpdDiffRR : Sum  Inputs=+-  OutDataTypeStr=single  AccumDataTypeStr=single
  Switch : Switch  Criteria=u2 > Threshold  OutDataTypeStr=single  SaturateOnIntegerOverflow=off  InputSameDT=off
  LSD_TrqRR : Outport  VectorParamsAs1DForOutWhenUnconnected=off
  wires:
  Add1/1 -> Switch/1  "LSDTrqRR"
  LSD_CtrlRR/1 -> Bus Selector/1
  Switch/1 -> LSD_TrqRR/1  "LSD_TrqRR"
  Bus Selector/3 -> Switch/2  "<LSD_EnableRR>"
  EDS_TrqRR/1 -> Add1/2, Switch/3
  PID Controller/1 -> Saturation1/1  "TrqModRR"
  Bus Selector/2 -> SpdDiffRR/2  "<MotSpdActlByrpmRR>"
  Demux/3 -> PID Controller/4  "D"
  Demux/2 -> PID Controller/3  "I"
  PID_Setting/1 -> Demux/1
  Demux/5 -> PID Controller/6  "PID_Reset"
  Gain/1 -> PID Controller/1  "SpdDiffRRScaled"
  Demux/4 -> PID Controller/5  "N"
  Bus Selector/1 -> SpdDiffRR/1  "<MotSpdRefByrpmRR>"
  Demux/1 -> PID Controller/2  "P"
  SpdDiffRR/1 -> Gain/1  "SpdDiffRR"
  Saturation1/1 -> Add1/1

== system VMC_14Dof_2024a/Subsystem1/Traction_Control/LimitedSlipDifferential/Subsystem ==
  LSD_Enable : Inport
  Controller_Setting : Inport  Port=2
  Bus Selector : BusSelector  OutputSignals=TC_Controller.TC_PID.TC_P,TC_Controller.TC_PID.TC_I,TC_Controller.TC_PID.TC_D
  Constant15 : Constant  Value=100  OutDataTypeStr=single  SampleTime=-1
  Data Type Conversion : DataTypeConversion  OutDataTypeStr=single  SaturateOnIntegerOverflow=off  RndMeth=Floor
  Demux : Demux
  Logical Operator1 : Logic  Operator=NAND  AllPortsSameDT=off  OutDataTypeStr=boolean
  Logical Operator2 : Logic  Operator=NAND  AllPortsSameDT=off  OutDataTypeStr=boolean
  Mux5 : Mux  Inputs=5
  Terminator : Terminator
  PID_Setting : Outport
  wires:
  Demux/4 -> Logical Operator1/2
  Demux/2 -> Logical Operator2/1
  Bus Selector/2 -> Mux5/2  "<TC_I>"
  Data Type Conversion/1 -> Mux5/5
  Mux5/1 -> PID_Setting/1  "PID_ParaFL"
  Constant15/1 -> Mux5/4  "N"
  Logical Operator1/1 -> Data Type Conversion/1
  Demux/3 -> Logical Operator2/2
  Demux/1 -> Logical Operator1/1
  Bus Selector/3 -> Mux5/3  "<TC_D>"
  LSD_Enable/1 -> Demux/1
  Bus Selector/1 -> Mux5/1  "<TC_P>"
  Logical Operator2/1 -> Terminator/1
  Controller_Setting/1 -> Bus Selector/1

== system VMC_14Dof_2024a/Subsystem1/Vehicle_State_Estimation/Tire_Force/Normal_Force ==
  m_FL_kg : Inport
  m_FR_kg : Inport  Port=2
  m_RL_kg : Inport  Port=3
  m_RR_kg : Inport  Port=4
  ax_mpss : Inport  Port=5
  ay_mpss : Inport  Port=6
  h_CoG_m : Inport  Port=7
  Wheelbase_m : Inport  Port=8
  Krf_Nmprad : Inport  Port=9
  Krr_Nmprad : Inport  Port=10
  Zrf_m : Inport  Port=11
  Zrr_m : Inport  Port=12
  tf_m : Inport  Port=13
  tr_m : Inport  Port=14
  lf_m : Inport  Port=15
  lr_m : Inport  Port=16
  ClA : Inport  Port=17
  rho : Inport  Port=18
  V_CoG_mps : Inport  Port=19
  Aero_Ratio : Inport  Port=20
  Normal_Force_Cal : MATLAB Function  TreatAsAtomicUnit=on
  Saturation{,1..3} (4 alike) : Saturate  UpperLimit=3000  LowerLimit=0
  Fz_FL_N : Outport
  Fz_FR_N : Outport  Port=2
  Fz_RL_N : Outport  Port=3
  Fz_RR_N : Outport  Port=4
  wires:
  m_FL_kg/1 -> Normal_Force_Cal/1(m_FL)
  m_FR_kg/1 -> Normal_Force_Cal/2(m_FR)
  m_RL_kg/1 -> Normal_Force_Cal/3(m_RL)
  m_RR_kg/1 -> Normal_Force_Cal/4(m_RR)
  ax_mpss/1 -> Normal_Force_Cal/5(ax)
  ay_mpss/1 -> Normal_Force_Cal/6(ay)
  h_CoG_m/1 -> Normal_Force_Cal/7(h_CoG)
  Wheelbase_m/1 -> Normal_Force_Cal/8(L)
  Krf_Nmprad/1 -> Normal_Force_Cal/9(Krf)
  Krr_Nmprad/1 -> Normal_Force_Cal/10(Krr)
  Zrf_m/1 -> Normal_Force_Cal/11(Zrf)
  Zrr_m/1 -> Normal_Force_Cal/12(Zrr)
  tf_m/1 -> Normal_Force_Cal/13(tf)
  tr_m/1 -> Normal_Force_Cal/14(tr)
  lf_m/1 -> Normal_Force_Cal/15(lf)
  lr_m/1 -> Normal_Force_Cal/16(lr)
  ClA/1 -> Normal_Force_Cal/17(ClA)
  rho/1 -> Normal_Force_Cal/18(rho)
  V_CoG_mps/1 -> Normal_Force_Cal/19(v)
  Aero_Ratio/1 -> Normal_Force_Cal/20(Aero_Ratio)
  Normal_Force_Cal/1(Fz_FL) -> Saturation/1
  Normal_Force_Cal/2(Fz_FR) -> Saturation1/1
  Normal_Force_Cal/3(Fz_RL) -> Saturation2/1
  Normal_Force_Cal/4(Fz_RR) -> Saturation3/1
  Saturation/1 -> Fz_FL_N/1
  Saturation1/1 -> Fz_FR_N/1
  Saturation2/1 -> Fz_RL_N/1
  Saturation3/1 -> Fz_RR_N/1

== system VMC_14Dof_2024a/Subsystem1/Vehicle_State_Estimation/Tractive_Regen_Torque/REG_Enable ==
  Brake_Demand_Pct : Inport  OutDataTypeStr=single
  MotorSpeed_Array_rpm : Inport  Port=2  OutDataTypeStr=single
  REG_Button_Bool : Inport  Port=3  OutDataTypeStr=boolean
  HV_Voltage_V : Inport  Port=4  OutDataTypeStr=single
  Compare To Constant1 : simulink/Logic and Bit Operations/Compare To Constant  relop=>  const=1500  OutDataTypeStr=boolean
  Compare To Constant2 : simulink/Logic and Bit Operations/Compare To Constant  relop=>  const=0  OutDataTypeStr=boolean
  Compare To Constant3 : simulink/Logic and Bit Operations/Compare To Constant  relop=<=  const=570  OutDataTypeStr=boolean
  Demux2 : Demux
  Logical Operator : Logic  Inputs=4  AllPortsSameDT=off  OutDataTypeStr=boolean
  Min : MinMax  Inputs=2  OutDataTypeStr=int16
  Terminator : Terminator
  Terminator1 : Terminator
  REG_Enable_Bool : Outport
  wires:
  Brake_Demand_Pct/1 -> Compare To Constant2/1
  Demux2/2 -> Terminator1/1
  HV_Voltage_V/1 -> Compare To Constant3/1
  Compare To Constant1/1 -> Logical Operator/1
  Demux2/1 -> Terminator/1
  REG_Button_Bool/1 -> Logical Operator/3
  Compare To Constant3/1 -> Logical Operator/4
  MotorSpeed_Array_rpm/1 -> Demux2/1
  Demux2/3 -> Min/1
  Min/1 -> Compare To Constant1/1
  Compare To Constant2/1 -> Logical Operator/2
  Demux2/4 -> Min/2
  Logical Operator/1 -> REG_Enable_Bool/1

== system VMC_14Dof_2024a/Subsystem1/YawRate_Controller/CalMz_FB/Avg_Wheel_Angle ==
  WheelAngle_Array_rad : Inport
  Constant : Constant  Value=2  OutDataTypeStr=single
  Demux : Demux
  Divide : Product  Inputs=*/  OutDataTypeStr=single
  Sum : Sum  OutDataTypeStr=single  AccumDataTypeStr=single
  Terminator : Terminator
  Terminator1 : Terminator
  Avg_WheelAngle_rad : Outport
  wires:
  Sum/1 -> Divide/1
  Constant/1 -> Divide/2
  Divide/1 -> Avg_WheelAngle_rad/1
  Demux/1 -> Sum/1
  Demux/2 -> Sum/2
  Demux/3 -> Terminator/1
  Demux/4 -> Terminator1/1
  WheelAngle_Array_rad/1 -> Demux/1

== system VMC_14Dof_2024a/Subsystem1/YawRate_Controller/CalMz_FB/TV_Reset ==
  Avg_WheelAngle_rad : Inport
  LateralAcceleration_mpss : Inport  Port=2
  Abs1 : Abs  OutDataTypeStr=single  SaturateOnIntegerOverflow=off
  Abs2 : Abs  OutDataTypeStr=single  SaturateOnIntegerOverflow=off
  Compare To Constant : simulink/Logic and Bit Operations/Compare To Constant  relop=<=  const=0.02  OutDataTypeStr=boolean
  Compare To Constant1 : simulink/Logic and Bit Operations/Compare To Constant  relop=<=  const=3  OutDataTypeStr=boolean
  Logical Operator : Logic  AllPortsSameDT=off  OutDataTypeStr=boolean
  TV_Reset : Outport
  wires:
  LateralAcceleration_mpss/1 -> Abs1/1
  Abs1/1 -> Compare To Constant1/1
  Logical Operator/1 -> TV_Reset/1  "TV_Reset"
  Compare To Constant/1 -> Logical Operator/1  "TV_Reset1"
  Compare To Constant1/1 -> Logical Operator/2  "TV_Reset2"
  Avg_WheelAngle_rad/1 -> Abs2/1
  Abs2/1 -> Compare To Constant/1

== system VMC_14Dof_2024a/Subsystem1/YawRate_Controller/CalcMzDes_FF/Avg_Wheel_Angle ==
  WheelAngle_Array_rad : Inport
  Constant : Constant  Value=2  OutDataTypeStr=single
  Demux : Demux
  Divide : Product  Inputs=*/  OutDataTypeStr=single
  Sum : Sum  OutDataTypeStr=single  AccumDataTypeStr=single
  Terminator : Terminator
  Terminator1 : Terminator
  Avg_WheelAngle_rad : Outport
  wires:
  Sum/1 -> Divide/1
  Constant/1 -> Divide/2
  Divide/1 -> Avg_WheelAngle_rad/1
  Demux/1 -> Sum/1
  Demux/2 -> Sum/2
  Demux/3 -> Terminator/1
  Demux/4 -> Terminator1/1
  WheelAngle_Array_rad/1 -> Demux/1

== system VMC_14Dof_2024a/Subsystem1/YawRate_Controller/CalcMzDes_FF/Integrator ==
  dx : Inport  PortDimensions=[5,1]
  Demux : Demux  Outputs=5
  Mux : Mux  Inputs=5
  integrator1 : Subsystem
  integrator2 : Subsystem
  integrator3 : Subsystem
  integrator4 : Subsystem
  integrator5 : Subsystem
  x : Outport  PortDimensions=[5,1]
  wires:
  dx/1 -> Demux/1
  Demux/1 -> integrator1/1(In)
  Demux/2 -> integrator2/1(In)
  Demux/3 -> integrator3/1(In)
  Demux/4 -> integrator4/1(In)
  Demux/5 -> integrator5/1(In)
  integrator1/1(Out) -> Mux/1
  integrator2/1(Out) -> Mux/2
  integrator3/1(Out) -> Mux/3
  integrator4/1(Out) -> Mux/4
  integrator5/1(Out) -> Mux/5
  Mux/1 -> x/1

== system VMC_14Dof_2024a/Subsystem/Body/Suspension_Z/fl/integrator1 ==
  In : Inport
  Add : Sum
  Add1 : Sum
  Constant : Constant  Value=Sampletime  OutDataTypeStr=single
  Constant1 : Constant  Value=0  OutDataTypeStr=single
  Delay1 : Delay  DelayLength=1  InitialCondition=0
  Divide : Product  Inputs=**
  Out : Outport  VectorParamsAs1DForOutWhenUnconnected=off
  wires:
  In/1 -> Divide/1
  Constant/1 -> Divide/2
  Divide/1 -> Add/1
  Delay1/1 -> Add/2, Add1/2
  Constant1/1 -> Add1/1
  Add/1 -> Delay1/1
  Add1/1 -> Out/1

== system VMC_14Dof_2024a/Subsystem/Body/Suspension_Z/fl/integrator2 ==
  In : Inport
  Add : Sum
  Add1 : Sum
  Constant : Constant  Value=Sampletime  OutDataTypeStr=single
  Constant1 : Constant  Value=0  OutDataTypeStr=single
  Delay1 : Delay  DelayLength=1  InitialCondition=0
  Divide : Product  Inputs=**
  Out : Outport  VectorParamsAs1DForOutWhenUnconnected=off
  wires:
  In/1 -> Divide/1
  Constant/1 -> Divide/2
  Divide/1 -> Add/1
  Delay1/1 -> Add/2, Add1/2
  Constant1/1 -> Add1/1
  Add/1 -> Delay1/1
  Add1/1 -> Out/1

== system VMC_14Dof_2024a/Subsystem/Body/Suspension_Z/fr/integrator1 ==
  In : Inport
  Add : Sum
  Add1 : Sum
  Constant : Constant  Value=Sampletime  OutDataTypeStr=single
  Constant1 : Constant  Value=0  OutDataTypeStr=single
  Delay1 : Delay  DelayLength=1  InitialCondition=0
  Divide : Product  Inputs=**
  Out : Outport  VectorParamsAs1DForOutWhenUnconnected=off
  wires:
  In/1 -> Divide/1
  Constant/1 -> Divide/2
  Divide/1 -> Add/1
  Delay1/1 -> Add/2, Add1/2
  Constant1/1 -> Add1/1
  Add/1 -> Delay1/1
  Add1/1 -> Out/1

== system VMC_14Dof_2024a/Subsystem/Body/Suspension_Z/fr/integrator2 ==
  In : Inport
  Add : Sum
  Add1 : Sum
  Constant : Constant  Value=Sampletime  OutDataTypeStr=single
  Constant1 : Constant  Value=0  OutDataTypeStr=single
  Delay1 : Delay  DelayLength=1  InitialCondition=0
  Divide : Product  Inputs=**
  Out : Outport  VectorParamsAs1DForOutWhenUnconnected=off
  wires:
  In/1 -> Divide/1
  Constant/1 -> Divide/2
  Divide/1 -> Add/1
  Delay1/1 -> Add/2, Add1/2
  Constant1/1 -> Add1/1
  Add/1 -> Delay1/1
  Add1/1 -> Out/1

== system VMC_14Dof_2024a/Subsystem/Body/Suspension_Z/rl/integrator1 ==
  In : Inport
  Add : Sum
  Add1 : Sum
  Constant : Constant  Value=Sampletime  OutDataTypeStr=single
  Constant1 : Constant  Value=0  OutDataTypeStr=single
  Delay1 : Delay  DelayLength=1  InitialCondition=0
  Divide : Product  Inputs=**
  Out : Outport  VectorParamsAs1DForOutWhenUnconnected=off
  wires:
  In/1 -> Divide/1
  Constant/1 -> Divide/2
  Divide/1 -> Add/1
  Delay1/1 -> Add/2, Add1/2
  Constant1/1 -> Add1/1
  Add/1 -> Delay1/1
  Add1/1 -> Out/1

== system VMC_14Dof_2024a/Subsystem/Body/Suspension_Z/rl/integrator2 ==
  In : Inport
  Add : Sum
  Add1 : Sum
  Constant : Constant  Value=Sampletime  OutDataTypeStr=single
  Constant1 : Constant  Value=0  OutDataTypeStr=single
  Delay1 : Delay  DelayLength=1  InitialCondition=0
  Divide : Product  Inputs=**
  Out : Outport  VectorParamsAs1DForOutWhenUnconnected=off
  wires:
  In/1 -> Divide/1
  Constant/1 -> Divide/2
  Divide/1 -> Add/1
  Delay1/1 -> Add/2, Add1/2
  Constant1/1 -> Add1/1
  Add/1 -> Delay1/1
  Add1/1 -> Out/1

== system VMC_14Dof_2024a/Subsystem/Body/Suspension_Z/rr/integrator1 ==
  In : Inport
  Add : Sum
  Add1 : Sum
  Constant : Constant  Value=Sampletime  OutDataTypeStr=single
  Constant1 : Constant  Value=0  OutDataTypeStr=single
  Delay1 : Delay  DelayLength=1  InitialCondition=0
  Divide : Product  Inputs=**
  Out : Outport  VectorParamsAs1DForOutWhenUnconnected=off
  wires:
  In/1 -> Divide/1
  Constant/1 -> Divide/2
  Divide/1 -> Add/1
  Delay1/1 -> Add/2, Add1/2
  Constant1/1 -> Add1/1
  Add/1 -> Delay1/1
  Add1/1 -> Out/1

== system VMC_14Dof_2024a/Subsystem/Body/Suspension_Z/rr/integrator2 ==
  In : Inport
  Add : Sum
  Add1 : Sum
  Constant : Constant  Value=Sampletime  OutDataTypeStr=single
  Constant1 : Constant  Value=0  OutDataTypeStr=single
  Delay1 : Delay  DelayLength=1  InitialCondition=0
  Divide : Product  Inputs=**
  Out : Outport  VectorParamsAs1DForOutWhenUnconnected=off
  wires:
  In/1 -> Divide/1
  Constant/1 -> Divide/2
  Divide/1 -> Add/1
  Delay1/1 -> Add/2, Add1/2
  Constant1/1 -> Add1/1
  Add/1 -> Delay1/1
  Add1/1 -> Out/1

== system VMC_14Dof_2024a/Subsystem/Body/Suspension_Z/zb_to_zs/integrator1 ==
  In : Inport
  Add : Sum
  Add1 : Sum
  Constant : Constant  Value=Sampletime  OutDataTypeStr=single
  Constant1 : Constant  Value=0  OutDataTypeStr=single
  Delay1 : Delay  DelayLength=1  InitialCondition=0
  Divide : Product  Inputs=**
  Out : Outport  VectorParamsAs1DForOutWhenUnconnected=off
  wires:
  In/1 -> Divide/1
  Constant/1 -> Divide/2
  Divide/1 -> Add/1
  Delay1/1 -> Add/2, Add1/2
  Constant1/1 -> Add1/1
  Add/1 -> Delay1/1
  Add1/1 -> Out/1

== system VMC_14Dof_2024a/Subsystem/Body/Suspension_Z/zb_to_zs/integrator2 ==
  In : Inport
  Add : Sum
  Add1 : Sum
  Constant : Constant  Value=Sampletime  OutDataTypeStr=single
  Constant1 : Constant  Value=0  OutDataTypeStr=single
  Delay1 : Delay  DelayLength=1  InitialCondition=0
  Divide : Product  Inputs=**
  Out : Outport  VectorParamsAs1DForOutWhenUnconnected=off
  wires:
  In/1 -> Divide/1
  Constant/1 -> Divide/2
  Divide/1 -> Add/1
  Delay1/1 -> Add/2, Add1/2
  Constant1/1 -> Add1/1
  Add/1 -> Delay1/1
  Add1/1 -> Out/1

== system VMC_14Dof_2024a/Subsystem/Body/Suspension_Z/zb_to_zs/integrator3 ==
  In : Inport
  Add : Sum
  Add1 : Sum
  Constant : Constant  Value=Sampletime  OutDataTypeStr=single
  Constant1 : Constant  Value=0  OutDataTypeStr=single
  Delay1 : Delay  DelayLength=1  InitialCondition=0
  Divide : Product  Inputs=**
  Out : Outport  VectorParamsAs1DForOutWhenUnconnected=off
  wires:
  In/1 -> Divide/1
  Constant/1 -> Divide/2
  Divide/1 -> Add/1
  Delay1/1 -> Add/2, Add1/2
  Constant1/1 -> Add1/1
  Add/1 -> Delay1/1
  Add1/1 -> Out/1
